simulink model "DiscretePIDAwFf"  (R2020b)
settings: Solver=FixedStepAuto  StartTime=0.0  StopTime=5  FixedStep=1e-4  RelTol=1e-3
undefined symbols (not defined in the file): daq, DiscIntNeverNeededParam, drv, est_par, gbox, io, mech, mld, mot, pid, rads2rpm, rpm2degs, sens, sim
libraries: simulink x1
settings Model: Creator=Utente  LastModifiedBy=Utente

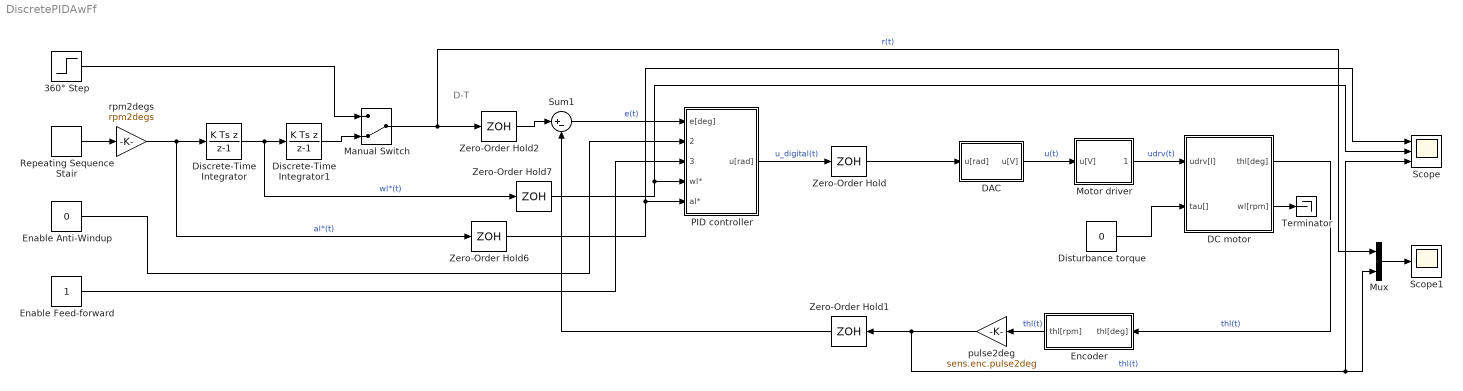
== system DiscretePIDAwFf ==
  note: D-T
  360° Step : Step  Time=0  After=360  SampleTime=0
  DAC : Subsystem
  DC motor : Subsystem
  Discrete-Time Integrator : DiscreteIntegrator  IntegratorMethod=Integration: Backward Euler  SampleTime=sim.T_samp  ICPrevOutput=DiscIntNeverNeededParam  ICPrevScaledInput=DiscIntNeverNeededParam
  Discrete-Time Integrator1 : DiscreteIntegrator  IntegratorMethod=Integration: Backward Euler  SampleTime=sim.T_samp  ICPrevOutput=DiscIntNeverNeededParam  ICPrevScaledInput=DiscIntNeverNeededParam
  Disturbance torque : Constant  Value=0
  Enable Anti-Windup : Constant  Value=0
  Enable Feed-forward : Constant
  Encoder : Subsystem
  Manual Switch : ManualSwitch  CurrentSetting=0
  Motor driver : Subsystem
  Mux : Mux  Inputs=2
  PID controller : Subsystem
  Repeating Sequence Stair : simulink/Sources/Repeating Sequence Stair  OutValues=[900 0 -900 -900 0 900].'  tsamp=0.5  OutMin=[]  OutMax=[]  OutDataTypeStr=double  OutputDataTypeScalingMode=double  OutDataType=fixdt(0,8)  ConRadixGroup=Best Precision: Vector-wise  OutScaling=2^-12
  Scope : Scope  NumInputPorts=3
  Scope1 : Scope
  Sum1 : Sum  Inputs=|+-
  Terminator : Terminator
  Zero-Order Hold{,1..2,6..7} (5 alike) : ZeroOrderHold  SampleTime=sim.T_samp
  pulse2deg : Gain  Gain=sens.enc.pulse2deg
  rpm2degs : Gain  Gain=rpm2degs
  wires:
  PID controller/1(u[rad]) -> Zero-Order Hold/1  "u_digital(t)"
  Discrete-Time Integrator1/1 -> Manual Switch/2
  Repeating Sequence Stair/1 -> rpm2degs/1
  rpm2degs/1 -> Discrete-Time Integrator/1, Zero-Order Hold6/1  "al*(t)"
  360° Step/1 -> Manual Switch/1
  Enable Feed-forward/1 -> PID controller/3(ff_enable)
  DC motor/1(thl[deg]) -> Encoder/1(thl[deg])  "thl(t)"
  Disturbance torque/1 -> DC motor/2(tau[])
  Manual Switch/1 -> Mux/1, Zero-Order Hold2/1  "r(t)"
  Sum1/1 -> PID controller/1(e[deg])  "e(t)"
  Enable Anti-Windup/1 -> PID controller/2(aw_enable)
  DC motor/2(wl[rpm]) -> Terminator/1
  Discrete-Time Integrator/1 -> Discrete-Time Integrator1/1, Zero-Order Hold7/1  "wl*(t)"
  Mux/1 -> Scope1/1
  DAC/1(u[V]) -> Motor driver/1(u[V])  "u(t)"
  Motor driver/1(udrv[I]) -> DC motor/1(udrv[I])  "udrv(t)"
  pulse2deg/1 -> Zero-Order Hold1/1, Scope/3, Mux/2  "thl(t)"
  Encoder/1(thl[rpm]) -> pulse2deg/1  "thl(t)"
  Zero-Order Hold/1 -> DAC/1(u[rad])
  Zero-Order Hold1/1 -> Sum1/2
  Zero-Order Hold2/1 -> Sum1/1
  Zero-Order Hold6/1 -> PID controller/5(al*), Scope/1
  Zero-Order Hold7/1 -> PID controller/4(wl*), Scope/2

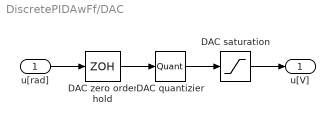
== system DiscretePIDAwFf/DAC ==
  u[rad] : Inport
  DAC quantizier : Quantizer  QuantizationInterval=daq.dac.q
  DAC saturation : Saturate  UpperLimit=daq.dac.vdd  LowerLimit=daq.dac.vss
  DAC zero order hold : ZeroOrderHold  SampleTime=daq.dac.T_s
  u[V] : Outport
  wires:
  DAC quantizier/1 -> DAC saturation/1
  DAC zero order hold/1 -> DAC quantizier/1
  DAC saturation/1 -> u[V]/1
  u[rad]/1 -> DAC zero order hold/1

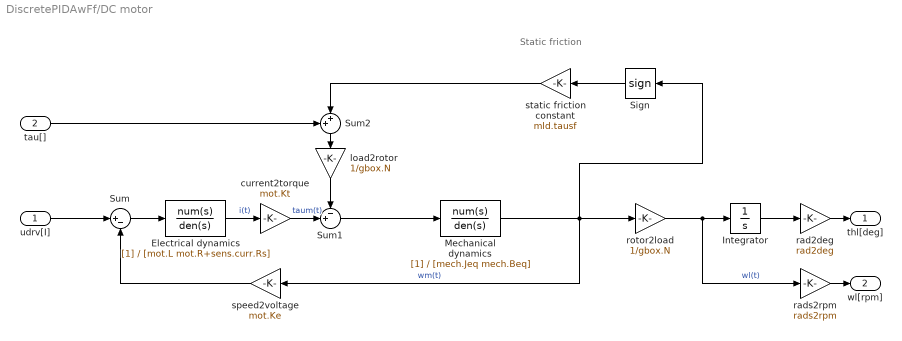
== system DiscretePIDAwFf/DC motor ==
  note: Static friction
  udrv[I] : Inport  Unit=V
  tau[] : Inport  Port=2  Unit=V
  Electrical dynamics : TransferFcn  Denominator=[mot.L mot.R+sens.curr.Rs]
  Integrator : Integrator
  Mechanical dynamics : TransferFcn  Denominator=[mech.Jeq mech.Beq]
  Sign : Signum  ZeroCross=off
  Sum : Sum  Inputs=|+-
  Sum1 : Sum  Inputs=-+|
  Sum2 : Sum  Inputs=++|
  current2torque : Gain  Gain=mot.Kt
  load2rotor : Gain  Gain=1/gbox.N
  rad2deg : Gain  Gain=rad2deg
  rads2rpm : Gain  Gain=rads2rpm
  rotor2load : Gain  Gain=1/gbox.N
  speed2voltage : Gain  Gain=mot.Ke
  static friction constant : Gain  Gain=mld.tausf
  thl[deg] : Outport  Unit=deg
  wl[rpm] : Outport  Port=2  Unit=rpm
  wires:
  load2rotor/1 -> Sum1/1
  Mechanical dynamics/1 -> Sign/1, rotor2load/1, speed2voltage/1  "wm(t)"
  Sign/1 -> static friction constant/1
  current2torque/1 -> Sum1/2  "taum(t)"
  Sum1/1 -> Mechanical dynamics/1
  speed2voltage/1 -> Sum/2
  rotor2load/1 -> rads2rpm/1, Integrator/1  "wl(t)"
  Electrical dynamics/1 -> current2torque/1  "i(t)"
  Integrator/1 -> rad2deg/1
  Sum/1 -> Electrical dynamics/1
  rads2rpm/1 -> wl[rpm]/1
  rad2deg/1 -> thl[deg]/1
  udrv[I]/1 -> Sum/1
  Sum2/1 -> load2rotor/1
  tau[]/1 -> Sum2/1
  static friction constant/1 -> Sum2/2

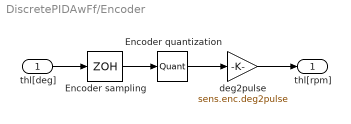
== system DiscretePIDAwFf/Encoder ==
  thl[deg] : Inport
  Encoder quantization : Quantizer  QuantizationInterval=sens.enc.q
  Encoder sampling : ZeroOrderHold  SampleTime=sens.enc.T_s
  deg2pulse : Gain  Gain=sens.enc.deg2pulse
  thl[rpm] : Outport
  wires:
  Encoder quantization/1 -> deg2pulse/1
  deg2pulse/1 -> thl[rpm]/1
  Encoder sampling/1 -> Encoder quantization/1
  thl[deg]/1 -> Encoder sampling/1

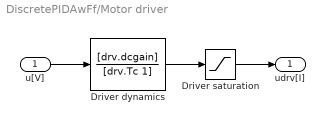
== system DiscretePIDAwFf/Motor driver ==
  u[V] : Inport
  Driver dynamics : TransferFcn  Numerator=[drv.dcgain]  Denominator=[drv.Tc 1]
  Driver saturation : Saturate  UpperLimit=drv.vp  LowerLimit=drv.vm
  udrv[I] : Outport
  wires:
  Driver saturation/1 -> udrv[I]/1
  Driver dynamics/1 -> Driver saturation/1
  u[V]/1 -> Driver dynamics/1

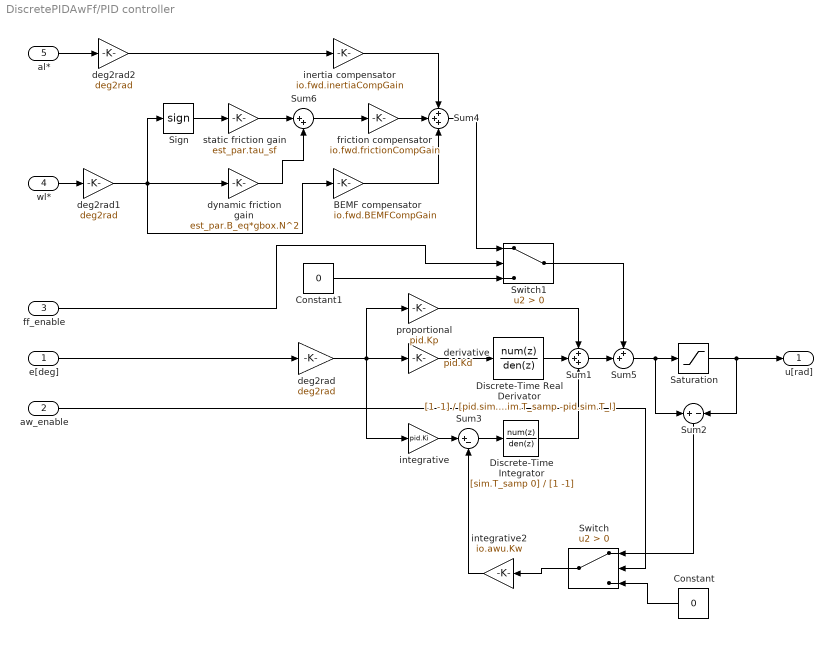
== system DiscretePIDAwFf/PID controller ==
  e[deg] : Inport  Unit=deg
  aw_enable : Inport  Port=2  Unit=deg
  ff_enable : Inport  Port=3  Unit=deg
  wl* : Inport  Port=4  Unit=deg
  al* : Inport  Port=5  Unit=deg
  BEMF compensator : Gain  Gain=io.fwd.BEMFCompGain
  Constant : Constant  Value=0
  Constant1 : Constant  Value=0
  Discrete-Time Integrator : DiscreteTransferFcn  Numerator=[sim.T_samp 0]  Denominator=[1 -1]  SampleTime=sim.T_samp
  Discrete-Time Real Derivator : DiscreteTransferFcn  Numerator=[1 -1]  Denominator=[pid.sim.T_l+sim.T_samp -pid.sim.T_l]  SampleTime=sim.T_samp
  Saturation : Saturate  UpperLimit=daq.dac.vdd  LowerLimit=daq.dac.vss
  Sign : Signum
  Sum1 : Sum  Inputs=+++
  Sum2 : Sum  Inputs=+|-
  Sum3 : Sum  Inputs=|+-
  Sum4 : Sum  Inputs=+++
  Sum5 : Sum  Inputs=++|
  Sum6 : Sum  Inputs=|++
  Switch : Switch  Criteria=u2 > Threshold
  Switch1 : Switch  Criteria=u2 > Threshold
  deg2rad : Gain  Gain=deg2rad
  deg2rad1 : Gain  Gain=deg2rad
  deg2rad2 : Gain  Gain=deg2rad
  derivative : Gain  Gain=pid.Kd
  dynamic friction gain : Gain  Gain=est_par.B_eq*gbox.N^2
  friction compensator : Gain  Gain=io.fwd.frictionCompGain
  inertia compensator : Gain  Gain=io.fwd.inertiaCompGain
  integrative : Gain  Gain=pid.Ki
  integrative2 : Gain  Gain=io.awu.Kw
  proportional : Gain  Gain=pid.Kp
  static friction gain : Gain  Gain=est_par.tau_sf
  u[rad] : Outport
  wires:
  e[deg]/1 -> deg2rad/1
  deg2rad1/1 -> BEMF compensator/1, Sign/1, dynamic friction gain/1
  deg2rad2/1 -> inertia compensator/1
  proportional/1 -> Sum1/1
  friction compensator/1 -> Sum4/2
  Constant1/1 -> Switch1/3
  integrative2/1 -> Sum3/2
  Switch1/1 -> Sum5/1
  Sign/1 -> static friction gain/1
  Discrete-Time Real Derivator/1 -> Sum1/2
  al*/1 -> deg2rad2/1
  wl*/1 -> deg2rad1/1
  Sum5/1 -> Saturation/1, Sum2/1
  Switch/1 -> integrative2/1
  Sum4/1 -> Switch1/1
  Saturation/1 -> Sum2/2, u[rad]/1
  Constant/1 -> Switch/3
  static friction gain/1 -> Sum6/1
  dynamic friction gain/1 -> Sum6/2
  ff_enable/1 -> Switch1/2
  integrative/1 -> Sum3/1
  Sum6/1 -> friction compensator/1
  deg2rad/1 -> integrative/1, derivative/1, proportional/1
  BEMF compensator/1 -> Sum4/3
  aw_enable/1 -> Switch/2
  Discrete-Time Integrator/1 -> Sum1/3
  Sum2/1 -> Switch/1
  inertia compensator/1 -> Sum4/1
  Sum1/1 -> Sum5/2
  derivative/1 -> Discrete-Time Real Derivator/1
  Sum3/1 -> Discrete-Time Integrator/1
